simulink model "buck_boost"  (R2024a)
settings: Solver=VariableStepAuto  StartTime=0.0  StopTime=10.0  RelTol=1e-3
values from neighbouring files (symbols this model uses):
  C = 0.0016    [buck_boost.mat]
  D = 0.6    [buck_boost.mat]
  f = 10000    [buck_boost.mat]
  L = 0.0003    [buck_boost.mat]
  R = 3.75    [buck_boost.mat]
  Vi = 10    [buck_boost.mat]
libraries: spsCurrentMeasurementLib x3, spsVoltageMeasurementLib x3, spsSeriesRLCBranchLib x3, spsDiodeLib x1, spsMosfetLib x1, spsDCVoltageSourceLib x1, sps_lib x1
settings Model: Creator=Anshuman  LastModifiedBy=Anshuman

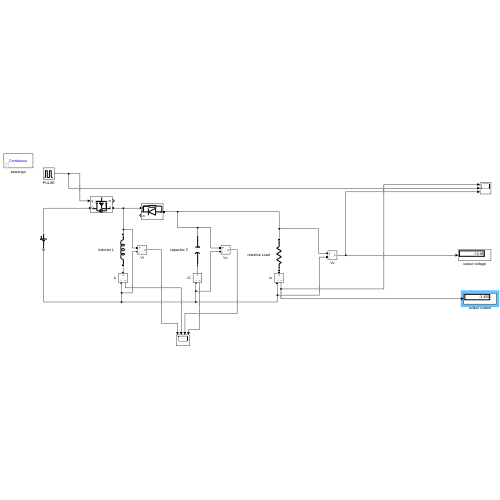
[thumbnail: Simulink's stored preview of the top-level diagram]
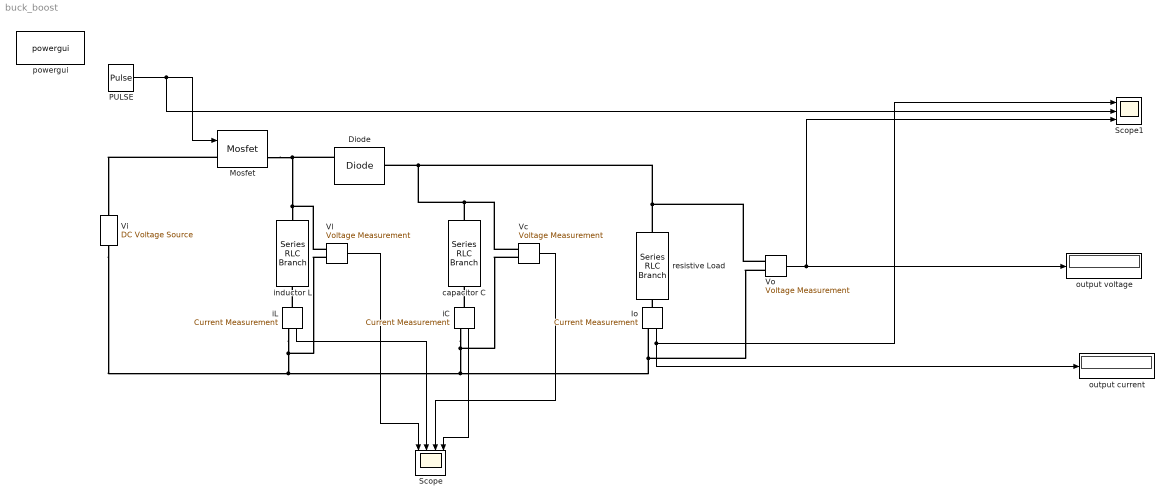
== system buck_boost ==
  Diode : spsDiodeLib/Diode  Ron=0.001  Lon=0  Vf=0.8  IC=0  UseSnubber=0  Rs=500  Cs=250e-9  Measurements=on
  Io : spsCurrentMeasurementLib/Current Measurement  PhasorSimulation=off  OutputType=Complex  PSBequivalent=0
  Mosfet : spsMosfetLib/Mosfet  Ron=0.1  Lon=0  Rd=0.01  Vfd=0  IC=0  Rs=1e5  Cs=inf  Measurements=on
  PULSE : DiscretePulseGenerator  PulseType=Time based  Period=1/f  PulseWidth=100*D
  Scope : Scope  NumInputPorts=4
  Scope1 : Scope  NumInputPorts=3
  Vc : spsVoltageMeasurementLib/Voltage Measurement  PhasorSimulation=off  OutputType=Complex  PSBequivalent=0
  Vi : spsDCVoltageSourceLib/DC Voltage Source  Amplitude=Vi  Measurements=None
  Vl : spsVoltageMeasurementLib/Voltage Measurement  PhasorSimulation=off  OutputType=Complex  PSBequivalent=0
  Vo : spsVoltageMeasurementLib/Voltage Measurement  PhasorSimulation=off  OutputType=Complex  PSBequivalent=0
  capacitor C : spsSeriesRLCBranchLib/Series RLC Branch  LConnTagsString=__new0  RConnTagsString=__new0  BranchType=C  Resistance=1  Inductance=1e-3  SetiL0=off  InitialCurrent=0  Capacitance=C  Setx0=off  InitialVoltage=0  Measurements=None
  iC : spsCurrentMeasurementLib/Current Measurement  PhasorSimulation=off  OutputType=Complex  PSBequivalent=0
  iL : spsCurrentMeasurementLib/Current Measurement  PhasorSimulation=off  OutputType=Complex  PSBequivalent=0
  inductor L : spsSeriesRLCBranchLib/Series RLC Branch  LConnTagsString=__new0  RConnTagsString=__new0  BranchType=L  Resistance=1  Inductance=L  SetiL0=off  InitialCurrent=0  Capacitance=1e-6  Setx0=off  InitialVoltage=0  Measurements=None
  output current : Display
  output voltage : Display
  powergui : sps_lib/powergui  Priority=1  SimulationMode=Continuous  SampleTime=50e-6  frequency=60  Iterations=50  frequencyindice=0  Pbase=100e6  ErrMax=1e-4  UnitsV=kV  UnitsW=MW  buscounter=0  FunctionMessages=off  echomessages=off  EnableUseOfTLC=off  CurrentSourceSwitches=off  DisableSnubberDevices=off  DisableRonSwitches=off  DisableVfSwitches=off  DisplayEquations=off  AutomaticDiscreteSolvers=off  SolverType=Tustin/Backward Euler (TBE)  Interpol=off  ExternalGateDelay=off  methode=off  Ts=100  x0status=blocks  SPID=on  SwTol=0  HookPort=off  NonlinearTolerance=1e-4  nMaxIteration=100  ContinueOnMaxIteration=off  RestoreLinks=warning  ResistiveCurrentMeasurement=off  Frange=[0:2:500]  Ylog=off  Xlog=on  ShowGrid=off  save=off  variable=ZData  structure=0  ZoomFFT=off  StartTime=0.0  cycles=1  DisplayStyle=1  fundamental=60  FreqAxis=off  MaxFrequency=1000  frequencyindicesteady=1  RmsSteady=1  display=off
  resistive Load : spsSeriesRLCBranchLib/Series RLC Branch  LConnTagsString=__new0  RConnTagsString=__new0  BranchType=R  Resistance=R  Inductance=1e-3  SetiL0=off  InitialCurrent=0  Capacitance=1e-6  Setx0=off  InitialVoltage=0  Measurements=None
  wires:
  PULSE/1 -> Mosfet/1, Scope1/2
  Vo/1 -> Scope1/3, output voltage/1
  Io/1 -> output current/1, Scope1/1
  Vl/1 -> Scope/1
  iL/1 -> Scope/2
  Vc/1 -> Scope/3
  iC/1 -> Scope/4
  connections:
  Mosfet/LConn1 -- Vi/RConn1
  Mosfet/RConn1 -- Diode/RConn1 -- Vl/LConn1 -- inductor L/LConn1
  capacitor C/LConn1 -- Vo/LConn1 -- resistive Load/LConn1 -- Diode/LConn1 -- Vc/LConn1
  iL/LConn1 -- inductor L/RConn1
  iC/LConn1 -- capacitor C/RConn1
  Io/LConn1 -- resistive Load/RConn1
  Vi/LConn1 -- Vl/LConn2 -- iL/RConn1 -- Vc/LConn2 -- iC/RConn1 -- Vo/LConn2 -- Io/RConn1
